simulink model "task1_2"  (R2019b)
settings: Solver=FixedStepDiscrete  StartTime=0.0  StopTime=100.0  FixedStep=0.001  RelTol=1e-3
InitFcn:
  | k = -1;
settings Model: Creator=linesLK  LastModifiedBy=linesLK

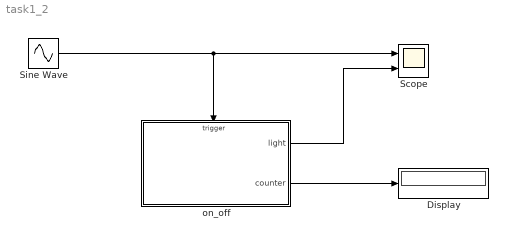
== system task1_2 ==
  Display : Display
  Scope : Scope  NumInputPorts=2
  Sine Wave : Sin  SampleTime=0
  on_off : Stateflow chart  BlockKeywords=__PRM__SERIALIZED__DATA__:Stateflow Chart,Stateflow Diagram  TreatAsAtomicUnit=on
  wires:
  Sine Wave/1 -> on_off/Trigger, Scope/1
  on_off/2(counter) -> Display/1
  on_off/1(light) -> Scope/2

== stateflow chart task1_2/on_off ==
  settings: executeAtInitialization=1
  state Power_on
    entry: light = k;
  state Power_off
    entry: light = 0;
  Power_on -> Power_off : Switch{counter=counter+1;}
  (default) -> Power_on
  Power_off -> Power_on : Switch{counter=counter+1;}
  data: light output double =0; counter output double =0; k parameter double
  events: Switch input RISING_EDGE_EVENT
